simulink model "StateSpace"  (R2021b)
settings: Solver=VariableStepAuto  StartTime=0.0  StopTime=10.0  RelTol=1e-3
undefined symbols (not defined in the file): AS, BFZ, BS
settings Model: Creator=jonih  LastModifiedBy=jonih

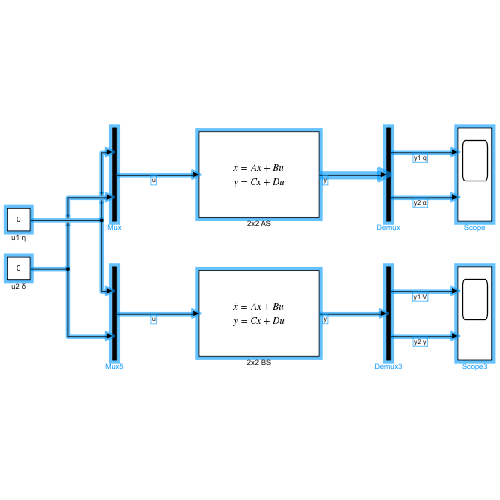
[thumbnail: Simulink's stored preview of the top-level diagram]
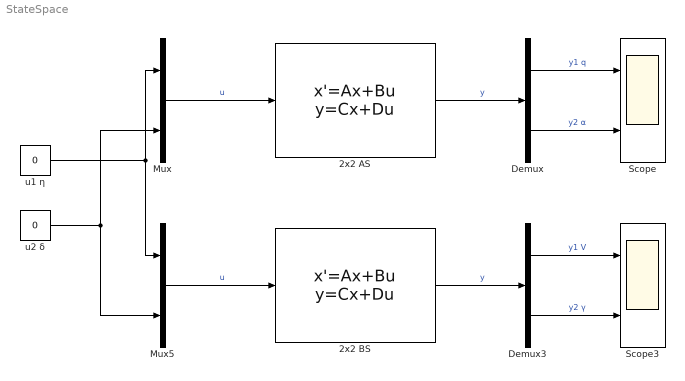
== system StateSpace ==
  2x2 AS : StateSpace  A=AS(1).A  B=AS(1).B  C=eye(2,2)  D=zeros(2,2)  InitialCondition=[0; BFZ(1).alpha]  ParameterTunability=Unconstrained  ContinuousStateAttributes={ 'q' , 'alpha' }
  2x2 BS : StateSpace  A=BS(1).A  B=BS(1).B  C=eye(2,2)  D=zeros(2,2)  InitialCondition=[0; BFZ(1).V]  ParameterTunability=Unconstrained  AllowTunableDMatrix=on  ContinuousStateAttributes={ 'V' , 'gamma' }
  Demux : Demux  Outputs=2
  Demux3 : Demux  Outputs=2
  Mux : Mux  Inputs=2
  Mux5 : Mux  Inputs=2
  Scope : Scope  NumInputPorts=2
  Scope3 : Scope  NumInputPorts=2
  u1 η : Constant  Value=0
  u2 δ : Constant  Value=0
  wires:
  u1 η/1 -> Mux/1, Mux5/1
  2x2 BS/1 -> Demux3/1  "y"
  u2 δ/1 -> Mux/2, Mux5/2
  Mux/1 -> 2x2 AS/1  "u"
  Demux3/1 -> Scope3/1  "y1 V"
  Mux5/1 -> 2x2 BS/1  "u"
  Demux/1 -> Scope/1  "y1 q"
  Demux3/2 -> Scope3/2  "y2 γ"
  Demux/2 -> Scope/2  "y2 α"
  2x2 AS/1 -> Demux/1  "y"
